simulink model "analyticSim"  (R2024b)
settings: Solver=VariableStepAuto  StartTime=0.0  StopTime=11  RelTol=1e-3
values from neighbouring files (symbols this model uses):
  K = 60    [freqAnal.m]
  numC = conv(numC, leadNumC)    [freqAnal.m]
settings Model: Creator=steve0gillet  LastModifiedBy=steve0gillet

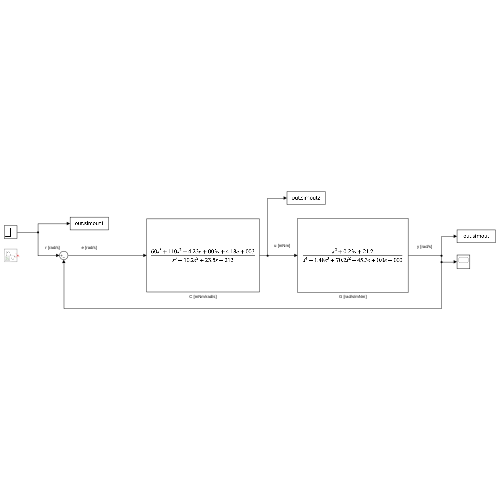
[thumbnail: Simulink's stored preview of the top-level diagram]
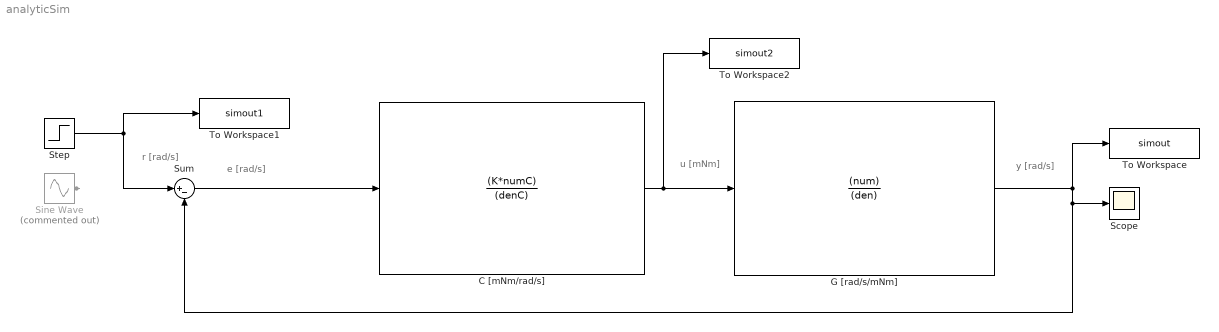
== system analyticSim ==
  note: u [mNm]
  note: y [rad/s]
  note: r [rad/s]
  note: e [rad/s]
  C [mNm/rad/s] : TransferFcn  Numerator=(K*numC)  Denominator=(denC)
  G [rad/s/mNm] : TransferFcn  Numerator=(num)  Denominator=(den)
  Scope : Scope
  Sine Wave : Sin  Commented=on  Amplitude=0.5  Frequency=pi  SampleTime=0
  Step : Step  After=0.5  SampleTime=0
  Sum : Sum  Inputs=|+-
  To Workspace : ToWorkspace  VariableName=simout  SaveFormat=Timeseries  SampleTime=-1
  To Workspace1 : ToWorkspace  VariableName=simout1  SaveFormat=Timeseries  SampleTime=-1
  To Workspace2 : ToWorkspace  VariableName=simout2  SaveFormat=Timeseries  SampleTime=-1
  wires:
  C [mNm/rad/s]/1 -> G [rad/s/mNm]/1, To Workspace2/1
  G [rad/s/mNm]/1 -> Sum/2, Scope/1, To Workspace/1
  Sum/1 -> C [mNm/rad/s]/1
  Step/1 -> To Workspace1/1, Sum/1
  Sine Wave/1 -> ?
